simulink model "mainModelDoeJF"  (R2025a)
(part 2 of 3)

  heatGenModule16/1 -> SPC16/1
  heatGenModule17/1 -> SPC17/1
  heatGenModule18/1 -> SPC18/1
  heatGenModule19/1 -> SPC19/1
  heatGenModule20/1 -> SPC20/1
  heatGenModule21/1 -> SPC21/1
  heatGenModule22/1 -> SPC22/1
  heatGenModule23/1 -> SPC23/1
  heatGenModule24/1 -> SPC24/1
  heatGenModule25/1 -> SPC25/1
  heatGenModule26/1 -> SPC26/1
  heatGenModule27/1 -> SPC27/1
  heatGenModule28/1 -> SPC28/1
  heatGenModule29/1 -> SPC29/1
  heatGenModule30/1 -> SPC30/1
  heatGenModule31/1 -> SPC31/1
  heatGenModule32/1 -> SPC32/1
  TempProbeBlock1/1 -> thermalToElectricalConverter1/1  "T1"
  TempProbeBlock2/1 -> thermalToElectricalConverter2/1  "T2"
  TempProbeBlock3/1 -> thermalToElectricalConverter3/1  "T3"
  TempProbeBlock4/1 -> thermalToElectricalConverter4/1  "T4"
  TempProbeBlock5/1 -> thermalToElectricalConverter5/1  "T5"
  TempProbeBlock6/1 -> thermalToElectricalConverter6/1  "T6"
  TempProbeBlock7/1 -> thermalToElectricalConverter7/1  "T7"
  TempProbeBlock8/1 -> thermalToElectricalConverter8/1  "T8"
  TempProbeBlock9/1 -> thermalToElectricalConverter9/1  "T9"
  TempProbeBlock10/1 -> thermalToElectricalConverter10/1  "T10"
  TempProbeBlock11/1 -> thermalToElectricalConverter11/1  "T11"
  TempProbeBlock12/1 -> thermalToElectricalConverter12/1  "T12"
  TempProbeBlock13/1 -> thermalToElectricalConverter13/1  "T13"
  TempProbeBlock14/1 -> thermalToElectricalConverter14/1  "T14"
  TempProbeBlock15/1 -> thermalToElectricalConverter15/1  "T15"
  TempProbeBlock16/1 -> thermalToElectricalConverter16/1  "T16"
  TempProbeBlock17/1 -> thermalToElectricalConverter17/1  "T17"
  TempProbeBlock18/1 -> thermalToElectricalConverter18/1  "T18"
  TempProbeBlock19/1 -> thermalToElectricalConverter19/1  "T19"
  TempProbeBlock20/1 -> thermalToElectricalConverter20/1  "T20"
  TempProbeBlock21/1 -> thermalToElectricalConverter21/1  "T21"
  TempProbeBlock22/1 -> thermalToElectricalConverter22/1  "T22"
  TempProbeBlock23/1 -> thermalToElectricalConverter23/1  "T23"
  TempProbeBlock24/1 -> thermalToElectricalConverter24/1  "T24"
  TempProbeBlock25/1 -> thermalToElectricalConverter25/1  "T25"
  TempProbeBlock26/1 -> thermalToElectricalConverter26/1  "T26"
  TempProbeBlock27/1 -> thermalToElectricalConverter27/1  "T27"
  TempProbeBlock28/1 -> thermalToElectricalConverter28/1  "T28"
  TempProbeBlock29/1 -> thermalToElectricalConverter29/1  "T29"
  TempProbeBlock30/1 -> thermalToElectricalConverter30/1  "T30"
  TempProbeBlock31/1 -> thermalToElectricalConverter31/1  "T31"
  TempProbeBlock32/1 -> thermalToElectricalConverter32/1  "T32"
  connections:
  Module1/RConn1 -- Module2/LConn2
  Module2/RConn1 -- Module3/LConn2
  Module3/RConn1 -- Module4/LConn2
  Module4/RConn1 -- Module5/LConn2
  Module5/RConn1 -- Module6/LConn2
  Module6/RConn1 -- Module7/LConn2
  Module7/RConn1 -- Module8/LConn2
  Module8/RConn1 -- Module9/LConn2
  Module9/RConn1 -- Module10/LConn2
  Module10/RConn1 -- Module11/LConn2
  Module11/RConn1 -- Module12/LConn2
  Module12/RConn1 -- Module13/LConn2
  Module13/RConn1 -- Module14/LConn2
  Module14/RConn1 -- Module15/LConn2
  Module15/RConn1 -- Module16/LConn2
  Module16/RConn1 -- Module17/LConn2
  Module17/RConn1 -- Module18/LConn2
  Module18/RConn1 -- Module19/LConn2
  Module19/RConn1 -- Module20/LConn2
  Module20/RConn1 -- Module21/LConn2
  Module21/RConn1 -- Module22/LConn2
  Module22/RConn1 -- Module23/LConn2
  Module23/RConn1 -- Module24/LConn2
  Module24/RConn1 -- Module25/LConn2
  Module25/RConn1 -- Module26/LConn2
  Module26/RConn1 -- Module27/LConn2
  Module27/RConn1 -- Module28/LConn2
  Module28/RConn1 -- Module29/LConn2
  Module29/RConn1 -- Module30/LConn2
  Module30/RConn1 -- Module31/LConn2
  Module31/RConn1 -- Module32/LConn2
  Constant1/RConn1 -- Cycler/LConn3
  currentProfiletoSimscape/RConn1 -- Cycler/LConn1
  Cycler/RConn1 -- Module1/LConn2
  Cycler/RConn2 -- SolverConfig/RConn1 -- Module32/RConn1 -- ElectricalRef/LConn1
  coolantSwitchConverter/RConn1 -- coolantSwitchMultiplier/LConn2
  AdvectiveCoeff/RConn1 -- coolantSwitchMultiplier/LConn1
  CoolantCPCC1/LConn2 -- ThermalMassCPCC29/LConn1 -- TR_TMCPCC29/LConn1 -- CoolantBC1/LConn3
  CoolantCPCC1/LConn3 -- CoolantCPCC2/LConn2 -- ThermalMassCPCC30/LConn1 -- TR_TMCPCC30/LConn1
  CoolantCPCC1/LConn1 -- coolantSwitchMultiplier/RConn1 -- CoolantCPCC2/LConn1 -- CoolantCPCC3/LConn1 -- CoolantCPCC4/LConn1 -- CoolantCPCC5/LConn1 -- CoolantCPCC6/LConn1 -- CoolantCPCC7/LConn1 -- CoolantCPCC8/LConn1 -- CoolantCPCC9/LConn1 -- CoolantCPCC10/LConn1 -- CoolantCPCC11/LConn1 -- CoolantCPCC12/LConn1 -- CoolantCPCC13/LConn1 -- CoolantCPCC14/LConn1 -- CoolantCPCC15/LConn1 -- CoolantCPCC16/LConn1 -- CoolantCPCC17/LConn1 -- CoolantCPCC18/LConn1 -- CoolantCPCC19/LConn1 -- CoolantCPCC20/LConn1 -- CoolantCPCC21/LConn1 -- CoolantCPCC22/LConn1 -- CoolantCPCC23/LConn1 -- CoolantCPCC24/LConn1 -- CoolantCPCC25/LConn1 -- CoolantCPCC26/LConn1 -- CoolantCPCC27/LConn1 -- CoolantCPCC28/LConn1 -- CoolantCPCC29/LConn1 -- CoolantCPCC30/LConn1 -- CoolantCPCC31/LConn1 -- CoolantCPHC1/LConn1 -- CoolantCPHC2/LConn1 -- CoolantCPHC3/LConn1 -- CoolantCPHC4/LConn1 -- CoolantCPHC5/LConn1 -- CoolantCPHC6/LConn1 -- CoolantCPHC7/LConn1 -- CoolantCPHC8/LConn1 -- CoolantCPHC9/LConn1 -- CoolantCPHC10/LConn1 -- CoolantCPHC11/LConn1 -- CoolantCPHC12/LConn1 -- CoolantCPHC13/LConn1 -- CoolantCPHC14/LConn1 -- CoolantCPHC15/LConn1 -- CoolantCPHC16/LConn1 -- CoolantCPHC17/LConn1 -- CoolantCPHC18/LConn1 -- CoolantCPHC19/LConn1 -- CoolantCPHC20/LConn1 -- CoolantCPHC21/LConn1 -- CoolantCPHC22/LConn1 -- CoolantCPHC23/LConn1 -- CoolantCPHC24/LConn1 -- CoolantCPHC25/LConn1 -- CoolantCPHC26/LConn1 -- CoolantCPHC27/LConn1 -- CoolantCPHC28/LConn1 -- CoolantCPHC29/LConn1 -- CoolantCPHC30/LConn1 -- CoolantCPHC31/LConn1 -- CoolanthotCoolConnect63/LConn1 -- CoolantBC1/LConn1 -- CoolantBC2/LConn1
  CoolantCPCC2/LConn3 -- CoolantCPCC3/LConn2 -- ThermalMassCPCC31/LConn1 -- TR_TMCPCC31/LConn1
  CoolantCPCC3/LConn3 -- CoolantCPCC4/LConn2 -- ThermalMassCPCC32/LConn1 -- TR_TMCPCC32/LConn1
  CoolantCPCC4/LConn3 -- CoolantCPCC5/LConn2 -- ThermalMassCPCC4/LConn1 -- TR_TMCPCC4/LConn1
  CoolantCPCC5/LConn3 -- CoolantCPCC6/LConn2 -- ThermalMassCPCC3/LConn1 -- TR_TMCPCC3/LConn1
  CoolantCPCC6/LConn3 -- CoolantCPCC7/LConn2 -- ThermalMassCPCC2/LConn1 -- TR_TMCPCC2/LConn1
  CoolantCPCC7/LConn3 -- CoolantCPCC29/LConn2 -- ThermalMassCPCC1/LConn1 -- TR_TMCPCC1/LConn1
  CoolantCPCC8/LConn2 -- ThermalMassCPCC5/LConn1 -- CoolantCPCC29/LConn3 -- TR_TMCPCC5/LConn1
  CoolantCPCC8/LConn3 -- CoolantCPCC9/LConn2 -- ThermalMassCPCC6/LConn1 -- TR_TMCPCC6/LConn1
  CoolantCPCC9/LConn3 -- CoolantCPCC10/LConn2 -- ThermalMassCPCC7/LConn1 -- TR_TMCPCC7/LConn1
  CoolantCPCC10/LConn3 -- CoolantCPCC11/LConn2 -- ThermalMassCPCC8/LConn1 -- TR_TMCPCC8/LConn1
  CoolantCPCC11/LConn3 -- CoolantCPCC12/LConn2 -- ThermalMassCPCC28/LConn1 -- TR_TMCPCC28/LConn1
  CoolantCPCC12/LConn3 -- CoolantCPCC13/LConn2 -- ThermalMassCPCC27/LConn1 -- TR_TMCPCC27/LConn1
  CoolantCPCC13/LConn3 -- CoolantCPCC14/LConn2 -- ThermalMassCPCC26/LConn1 -- TR_TMCPCC26/LConn1
  CoolantCPCC14/LConn3 -- CoolantCPCC30/LConn2 -- ThermalMassCPCC25/LConn1 -- TR_TMCPCC25/LConn1
  CoolantCPCC15/LConn2 -- ThermalMassCPCC21/LConn1 -- CoolantCPCC30/LConn3 -- TR_TMCPCC21/LConn1
  CoolantCPCC15/LConn3 -- CoolantCPCC16/LConn2 -- ThermalMassCPCC22/LConn1 -- TR_TMCPCC22/LConn1
  CoolantCPCC16/LConn3 -- CoolantCPCC17/LConn2 -- ThermalMassCPCC23/LConn1 -- TR_TMCPCC23/LConn1
  CoolantCPCC17/LConn3 -- CoolantCPCC18/LConn2 -- ThermalMassCPCC24/LConn1 -- TR_TMCPCC24/LConn1
  CoolantCPCC18/LConn3 -- CoolantCPCC19/LConn2 -- ThermalMassCPCC12/LConn1 -- TR_TMCPCC12/LConn1
  CoolantCPCC19/LConn3 -- CoolantCPCC20/LConn2 -- ThermalMassCPCC11/LConn1 -- TR_TMCPCC11/LConn1
  CoolantCPCC20/LConn3 -- CoolantCPCC21/LConn2 -- ThermalMassCPCC10/LConn1 -- TR_TMCPCC10/LConn1
  CoolantCPCC21/LConn3 -- CoolantCPCC31/LConn2 -- ThermalMassCPCC9/LConn1 -- TR_TMCPCC9/LConn1
  CoolantCPCC22/LConn2 -- ThermalMassCPCC13/LConn1 -- CoolantCPCC31/LConn3 -- TR_TMCPCC13/LConn1
  CoolantCPCC22/LConn3 -- CoolantCPCC23/LConn2 -- ThermalMassCPCC14/LConn1 -- TR_TMCPCC14/LConn1
  CoolantCPCC23/LConn3 -- CoolantCPCC24/LConn2 -- ThermalMassCPCC15/LConn1 -- TR_TMCPCC15/LConn1
  CoolantCPCC24/LConn3 -- CoolantCPCC25/LConn2 -- ThermalMassCPCC16/LConn1 -- TR_TMCPCC16/LConn1
  CoolantCPCC25/LConn3 -- CoolantCPCC26/LConn2 -- ThermalMassCPCC20/LConn1 -- TR_TMCPCC20/LConn1
  CoolantCPCC26/LConn3 -- CoolantCPCC27/LConn2 -- ThermalMassCPCC19/LConn1 -- TR_TMCPCC19/LConn1
  CoolantCPCC27/LConn3 -- CoolantCPCC28/LConn2 -- ThermalMassCPCC18/LConn1 -- TR_TMCPCC18/LConn1
  CoolantCPCC28/LConn3 -- CoolanthotCoolConnect63/LConn2 -- ThermalMassCPCC17/LConn1 -- TR_TMCPCC17/LConn1
  CoolantCPHC1/LConn3 -- ThermalMassCPHC29/LConn1 -- TR_TMCPHC29/LConn1 -- CoolantBC2/LConn2
  CoolantCPHC1/LConn2 -- CoolantCPHC2/LConn3 -- ThermalMassCPHC30/LConn1 -- TR_TMCPHC30/LConn1
  CoolantCPHC2/LConn2 -- CoolantCPHC3/LConn3 -- ThermalMassCPHC31/LConn1 -- TR_TMCPHC31/LConn1
  CoolantCPHC3/LConn2 -- CoolantCPHC4/LConn3 -- ThermalMassCPHC32/LConn1 -- TR_TMCPHC32/LConn1
  CoolantCPHC4/LConn2 -- CoolantCPHC5/LConn3 -- ThermalMassCPHC4/LConn1 -- TR_TMCPHC4/LConn1
  CoolantCPHC5/LConn2 -- CoolantCPHC6/LConn3 -- ThermalMassCPHC3/LConn1 -- TR_TMCPHC3/LConn1
  CoolantCPHC6/LConn2 -- CoolantCPHC7/LConn3 -- ThermalMassCPHC2/LConn1 -- TR_TMCPHC2/LConn1
  CoolantCPHC7/LConn2 -- CoolantCPHC29/LConn3 -- ThermalMassCPHC1/LConn1 -- TR_TMCPHC1/LConn1
  CoolantCPHC8/LConn3 -- ThermalMassCPHC5/LConn1 -- CoolantCPHC29/LConn2 -- TR_TMCPHC5/LConn1
  CoolantCPHC8/LConn2 -- CoolantCPHC9/LConn3 -- ThermalMassCPHC6/LConn1 -- TR_TMCPHC6/LConn1
  CoolantCPHC9/LConn2 -- CoolantCPHC10/LConn3 -- ThermalMassCPHC7/LConn1 -- TR_TMCPHC7/LConn1
  CoolantCPHC10/LConn2 -- CoolantCPHC11/LConn3 -- ThermalMassCPHC8/LConn1 -- TR_TMCPHC8/LConn1
  CoolantCPHC11/LConn2 -- CoolantCPHC12/LConn3 -- ThermalMassCPHC28/LConn1 -- TR_TMCPHC28/LConn1
  CoolantCPHC12/LConn2 -- CoolantCPHC13/LConn3 -- ThermalMassCPHC27/LConn1 -- TR_TMCPHC27/LConn1
  CoolantCPHC13/LConn2 -- CoolantCPHC14/LConn3 -- ThermalMassCPHC26/LConn1 -- TR_TMCPHC26/LConn1
  CoolantCPHC14/LConn2 -- CoolantCPHC30/LConn3 -- ThermalMassCPHC25/LConn1 -- TR_TMCPHC25/LConn1
  CoolantCPHC15/LConn3 -- ThermalMassCPHC21/LConn1 -- CoolantCPHC30/LConn2 -- TR_TMCPHC21/LConn1
  CoolantCPHC15/LConn2 -- CoolantCPHC16/LConn3 -- ThermalMassCPHC22/LConn1 -- TR_TMCPHC22/LConn1
  CoolantCPHC16/LConn2 -- CoolantCPHC17/LConn3 -- ThermalMassCPHC23/LConn1 -- TR_TMCPHC23/LConn1
  CoolantCPHC17/LConn2 -- CoolantCPHC18/LConn3 -- ThermalMassCPHC24/LConn1 -- TR_TMCPHC24/LConn1
  CoolantCPHC18/LConn2 -- CoolantCPHC19/LConn3 -- ThermalMassCPHC12/LConn1 -- TR_TMCPHC12/LConn1
  CoolantCPHC19/LConn2 -- CoolantCPHC20/LConn3 -- ThermalMassCPHC11/LConn1 -- TR_TMCPHC11/LConn1
  CoolantCPHC20/LConn2 -- CoolantCPHC21/LConn3 -- ThermalMassCPHC10/LConn1 -- TR_TMCPHC10/LConn1
  CoolantCPHC21/LConn2 -- CoolantCPHC31/LConn3 -- ThermalMassCPHC9/LConn1 -- TR_TMCPHC9/LConn1
  CoolantCPHC22/LConn3 -- ThermalMassCPHC13/LConn1 -- CoolantCPHC31/LConn2 -- TR_TMCPHC13/LConn1
  CoolantCPHC22/LConn2 -- CoolantCPHC23/LConn3 -- ThermalMassCPHC14/LConn1 -- TR_TMCPHC14/LConn1
  CoolantCPHC23/LConn2 -- CoolantCPHC24/LConn3 -- ThermalMassCPHC15/LConn1 -- TR_TMCPHC15/LConn1
  CoolantCPHC24/LConn2 -- CoolantCPHC25/LConn3 -- ThermalMassCPHC16/LConn1 -- TR_TMCPHC16/LConn1
  CoolantCPHC25/LConn2 -- CoolantCPHC26/LConn3 -- ThermalMassCPHC20/LConn1 -- TR_TMCPHC20/LConn1
  CoolantCPHC26/LConn2 -- CoolantCPHC27/LConn3 -- ThermalMassCPHC19/LConn1 -- TR_TMCPHC19/LConn1
  CoolantCPHC27/LConn2 -- CoolantCPHC28/LConn3 -- ThermalMassCPHC18/LConn1 -- TR_TMCPHC18/LConn1
  CoolantCPHC28/LConn2 -- CoolanthotCoolConnect63/LConn3 -- ThermalMassCPHC17/LConn1 -- TR_TMCPHC17/LConn1
  TR_TMCPCC1/RConn1 -- TR_TMCPHC1/RConn1 -- TR_MA1/RConn1 -- ThermalMassBatteries1/LConn1 -- heat1/LConn1
  TR_TMCPCC2/RConn1 -- TR_TMCPHC2/RConn1 -- TR_MA2/RConn1 -- ThermalMassBatteries2/LConn1 -- heat2/LConn1
  TR_TMCPCC3/RConn1 -- TR_TMCPHC3/RConn1 -- TR_MA3/RConn1 -- ThermalMassBatteries3/LConn1 -- heat3/LConn1
  TR_TMCPCC4/RConn1 -- TR_TMCPHC4/RConn1 -- TR_MA4/RConn1 -- ThermalMassBatteries4/LConn1 -- heat4/LConn1
  TR_TMCPCC5/RConn1 -- TR_TMCPHC5/RConn1 -- TR_MA5/RConn1 -- ThermalMassBatteries5/LConn1 -- heat5/LConn1
  TR_TMCPCC6/RConn1 -- TR_TMCPHC6/RConn1 -- TR_MA6/RConn1 -- ThermalMassBatteries6/LConn1 -- heat6/LConn1
  TR_TMCPCC7/RConn1 -- TR_TMCPHC7/RConn1 -- TR_MA7/RConn1 -- ThermalMassBatteries7/LConn1 -- heat7/LConn1
  TR_TMCPCC8/RConn1 -- TR_TMCPHC8/RConn1 -- TR_MA8/RConn1 -- ThermalMassBatteries8/LConn1 -- heat8/LConn1
  TR_TMCPCC9/RConn1 -- TR_TMCPHC9/RConn1 -- TR_MA9/RConn1 -- ThermalMassBatteries9/LConn1 -- heat9/LConn1
  TR_TMCPCC10/RConn1 -- TR_TMCPHC10/RConn1 -- TR_MA10/RConn1 -- ThermalMassBatteries10/LConn1 -- heat10/LConn1
  TR_TMCPCC11/RConn1 -- TR_TMCPHC11/RConn1 -- TR_MA11/RConn1 -- ThermalMassBatteries11/LConn1 -- heat11/LConn1
  TR_TMCPCC12/RConn1 -- TR_TMCPHC12/RConn1 -- TR_MA12/RConn1 -- ThermalMassBatteries12/LConn1 -- heat12/LConn1
  TR_TMCPCC13/RConn1 -- TR_TMCPHC13/RConn1 -- TR_MA13/RConn1 -- ThermalMassBatteries13/LConn1 -- heat13/LConn1
  TR_TMCPCC14/RConn1 -- TR_TMCPHC14/RConn1 -- TR_MA14/RConn1 -- ThermalMassBatteries14/LConn1 -- heat14/LConn1
  TR_TMCPCC15/RConn1 -- TR_TMCPHC15/RConn1 -- TR_MA15/RConn1 -- ThermalMassBatteries15/LConn1 -- heat15/LConn1
  TR_TMCPCC16/RConn1 -- TR_TMCPHC16/RConn1 -- TR_MA16/RConn1 -- ThermalMassBatteries16/LConn1 -- heat16/LConn1
  TR_TMCPCC17/RConn1 -- TR_TMCPHC17/RConn1 -- TR_MA17/RConn1 -- ThermalMassBatteries17/LConn1 -- heat17/LConn1
  TR_TMCPCC18/RConn1 -- TR_TMCPHC18/RConn1 -- TR_MA18/RConn1 -- ThermalMassBatteries18/LConn1 -- heat18/LConn1
  TR_TMCPCC19/RConn1 -- TR_TMCPHC19/RConn1 -- TR_MA19/RConn1 -- ThermalMassBatteries19/LConn1 -- heat19/LConn1
  TR_TMCPCC20/RConn1 -- TR_TMCPHC20/RConn1 -- TR_MA20/RConn1 -- ThermalMassBatteries20/LConn1 -- heat20/LConn1
  TR_TMCPCC21/RConn1 -- TR_TMCPHC21/RConn1 -- TR_MA21/RConn1 -- ThermalMassBatteries21/LConn1 -- heat21/LConn1
  TR_TMCPCC22/RConn1 -- TR_TMCPHC22/RConn1 -- TR_MA22/RConn1 -- ThermalMassBatteries22/LConn1 -- heat22/LConn1
  TR_TMCPCC23/RConn1 -- TR_TMCPHC23/RConn1 -- TR_MA23/RConn1 -- ThermalMassBatteries23/LConn1 -- heat23/LConn1
  TR_TMCPCC24/RConn1 -- TR_TMCPHC24/RConn1 -- TR_MA24/RConn1 -- ThermalMassBatteries24/LConn1 -- heat24/LConn1
  TR_TMCPCC25/RConn1 -- TR_TMCPHC25/RConn1 -- TR_MA25/RConn1 -- ThermalMassBatteries25/LConn1 -- heat25/LConn1
  TR_TMCPCC26/RConn1 -- TR_TMCPHC26/RConn1 -- TR_MA26/RConn1 -- ThermalMassBatteries26/LConn1 -- heat26/LConn1
  TR_TMCPCC27/RConn1 -- TR_TMCPHC27/RConn1 -- TR_MA27/RConn1 -- ThermalMassBatteries27/LConn1 -- heat27/LConn1
  TR_TMCPCC28/RConn1 -- TR_TMCPHC28/RConn1 -- TR_MA28/RConn1 -- ThermalMassBatteries28/LConn1 -- heat28/LConn1
  TR_TMCPCC29/RConn1 -- TR_TMCPHC29/RConn1 -- TR_MA29/RConn1 -- ThermalMassBatteries29/LConn1 -- heat29/LConn1
  TR_TMCPCC30/RConn1 -- TR_TMCPHC30/RConn1 -- TR_MA30/RConn1 -- ThermalMassBatteries30/LConn1 -- heat30/LConn1
  TR_TMCPCC31/RConn1 -- TR_TMCPHC31/RConn1 -- TR_MA31/RConn1 -- ThermalMassBatteries31/LConn1 -- heat31/LConn1
  TR_TMCPCC32/RConn1 -- TR_TMCPHC32/RConn1 -- TR_MA32/RConn1 -- ThermalMassBatteries32/LConn1 -- heat32/LConn1
  TempSource/RConn2 -- ThermalReference/LConn1 -- heat1/RConn2 -- heat2/RConn2 -- heat3/RConn2 -- heat4/RConn2 -- heat5/RConn2 -- heat6/RConn2 -- heat7/RConn2 -- heat8/RConn2 -- heat9/RConn2 -- heat10/RConn2 -- heat11/RConn2 -- heat12/RConn2 -- heat13/RConn2 -- heat14/RConn2 -- heat15/RConn2 -- heat16/RConn2 -- heat17/RConn2 -- heat18/RConn2 -- heat19/RConn2 -- heat20/RConn2 -- heat21/RConn2 -- heat22/RConn2 -- heat23/RConn2 -- heat24/RConn2 -- heat25/RConn2 -- heat26/RConn2 -- heat27/RConn2 -- heat28/RConn2 -- heat29/RConn2 -- heat30/RConn2 -- heat31/RConn2 -- heat32/RConn2 -- ThermalSolverConfig/RConn1
  ConstantTemp/RConn1 -- TempSource/RConn1
  TR_MA1/LConn1 -- TempSource/LConn1 -- TR_MA2/LConn1 -- TR_MA3/LConn1 -- TR_MA4/LConn1 -- TR_MA5/LConn1 -- TR_MA6/LConn1 -- TR_MA7/LConn1 -- TR_MA8/LConn1 -- TR_MA9/LConn1 -- TR_MA10/LConn1 -- TR_MA11/LConn1 -- TR_MA12/LConn1 -- TR_MA13/LConn1 -- TR_MA14/LConn1 -- TR_MA15/LConn1 -- TR_MA16/LConn1 -- TR_MA17/LConn1 -- TR_MA18/LConn1 -- TR_MA19/LConn1 -- TR_MA20/LConn1 -- TR_MA21/LConn1 -- TR_MA22/LConn1 -- TR_MA23/LConn1 -- TR_MA24/LConn1 -- TR_MA25/LConn1 -- TR_MA26/LConn1 -- TR_MA27/LConn1 -- TR_MA28/LConn1 -- TR_MA29/LConn1 -- TR_MA30/LConn1 -- TR_MA31/LConn1 -- TR_MA32/LConn1
  CoolantTempSource/LConn1 -- CoolantBC1/LConn2 -- CoolantBC2/LConn3
  SPC1/RConn1 -- heat1/RConn1
  SPC2/RConn1 -- heat2/RConn1
  SPC3/RConn1 -- heat3/RConn1
  SPC4/RConn1 -- heat4/RConn1
  SPC5/RConn1 -- heat5/RConn1
  SPC6/RConn1 -- heat6/RConn1
  SPC7/RConn1 -- heat7/RConn1
  SPC8/RConn1 -- heat8/RConn1
  SPC9/RConn1 -- heat9/RConn1
  SPC10/RConn1 -- heat10/RConn1
  SPC11/RConn1 -- heat11/RConn1
  SPC12/RConn1 -- heat12/RConn1
  SPC13/RConn1 -- heat13/RConn1
  SPC14/RConn1 -- heat14/RConn1
  SPC15/RConn1 -- heat15/RConn1
  SPC16/RConn1 -- heat16/RConn1
  SPC17/RConn1 -- heat17/RConn1
  SPC18/RConn1 -- heat18/RConn1
  SPC19/RConn1 -- heat19/RConn1
  SPC20/RConn1 -- heat20/RConn1
  SPC21/RConn1 -- heat21/RConn1
  SPC22/RConn1 -- heat22/RConn1
  SPC23/RConn1 -- heat23/RConn1
  SPC24/RConn1 -- heat24/RConn1
  SPC25/RConn1 -- heat25/RConn1
  SPC26/RConn1 -- heat26/RConn1
  SPC27/RConn1 -- heat27/RConn1
  SPC28/RConn1 -- heat28/RConn1
  SPC29/RConn1 -- heat29/RConn1
  SPC30/RConn1 -- heat30/RConn1
  SPC31/RConn1 -- heat31/RConn1
  SPC32/RConn1 -- heat32/RConn1
  tempSource1/RConn2 -- ThermalReferenceInElectricalModel/LConn1 -- tempSource2/RConn2 -- tempSource3/RConn2 -- tempSource4/RConn2 -- tempSource5/RConn2 -- tempSource6/RConn2 -- tempSource7/RConn2 -- tempSource8/RConn2 -- tempSource9/RConn2 -- tempSource10/RConn2 -- tempSource11/RConn2 -- tempSource12/RConn2 -- tempSource13/RConn2 -- tempSource14/RConn2 -- tempSource15/RConn2 -- tempSource16/RConn2 -- tempSource17/RConn2 -- tempSource18/RConn2 -- tempSource19/RConn2 -- tempSource20/RConn2 -- tempSource21/RConn2 -- tempSource22/RConn2 -- tempSource23/RConn2 -- tempSource24/RConn2 -- tempSource25/RConn2 -- tempSource26/RConn2 -- tempSource27/RConn2 -- tempSource28/RConn2 -- tempSource29/RConn2 -- tempSource30/RConn2 -- tempSource31/RConn2 -- tempSource32/RConn2
  tempSource1/LConn1 -- Module1/LConn1
  thermalToElectricalConverter1/RConn1 -- tempSource1/RConn1
  tempSource2/LConn1 -- Module2/LConn1
  thermalToElectricalConverter2/RConn1 -- tempSource2/RConn1
  tempSource3/LConn1 -- Module3/LConn1
  thermalToElectricalConverter3/RConn1 -- tempSource3/RConn1
  tempSource4/LConn1 -- Module4/LConn1
  thermalToElectricalConverter4/RConn1 -- tempSource4/RConn1
  tempSource5/LConn1 -- Module5/LConn1
  thermalToElectricalConverter5/RConn1 -- tempSource5/RConn1
  tempSource6/LConn1 -- Module6/LConn1
  thermalToElectricalConverter6/RConn1 -- tempSource6/RConn1
  tempSource7/LConn1 -- Module7/LConn1
  thermalToElectricalConverter7/RConn1 -- tempSource7/RConn1
  tempSource8/LConn1 -- Module8/LConn1
  thermalToElectricalConverter8/RConn1 -- tempSource8/RConn1
  tempSource9/LConn1 -- Module9/LConn1
  thermalToElectricalConverter9/RConn1 -- tempSource9/RConn1
  tempSource10/LConn1 -- Module10/LConn1
  thermalToElectricalConverter10/RConn1 -- tempSource10/RConn1
  tempSource11/LConn1 -- Module11/LConn1
  thermalToElectricalConverter11/RConn1 -- tempSource11/RConn1
  tempSource12/LConn1 -- Module12/LConn1
  thermalToElectricalConverter12/RConn1 -- tempSource12/RConn1
  tempSource13/LConn1 -- Module13/LConn1
  thermalToElectricalConverter13/RConn1 -- tempSource13/RConn1
  tempSource14/LConn1 -- Module14/LConn1
  thermalToElectricalConverter14/RConn1 -- tempSource14/RConn1
  tempSource15/LConn1 -- Module15/LConn1
  thermalToElectricalConverter15/RConn1 -- tempSource15/RConn1
  tempSource16/LConn1 -- Module16/LConn1
  thermalToElectricalConverter16/RConn1 -- tempSource16/RConn1
  tempSource17/LConn1 -- Module17/LConn1
  thermalToElectricalConverter17/RConn1 -- tempSource17/RConn1
  tempSource18/LConn1 -- Module18/LConn1
  thermalToElectricalConverter18/RConn1 -- tempSource18/RConn1
  tempSource19/LConn1 -- Module19/LConn1
  thermalToElectricalConverter19/RConn1 -- tempSource19/RConn1
  tempSource20/LConn1 -- Module20/LConn1
  thermalToElectricalConverter20/RConn1 -- tempSource20/RConn1
  tempSource21/LConn1 -- Module21/LConn1
  thermalToElectricalConverter21/RConn1 -- tempSource21/RConn1
  tempSource22/LConn1 -- Module22/LConn1
  thermalToElectricalConverter22/RConn1 -- tempSource22/RConn1
  tempSource23/LConn1 -- Module23/LConn1
  thermalToElectricalConverter23/RConn1 -- tempSource23/RConn1
  tempSource24/LConn1 -- Module24/LConn1
  thermalToElectricalConverter24/RConn1 -- tempSource24/RConn1
  tempSource25/LConn1 -- Module25/LConn1
  thermalToElectricalConverter25/RConn1 -- tempSource25/RConn1
  tempSource26/LConn1 -- Module26/LConn1
  thermalToElectricalConverter26/RConn1 -- tempSource26/RConn1
  tempSource27/LConn1 -- Module27/LConn1
  thermalToElectricalConverter27/RConn1 -- tempSource27/RConn1
  tempSource28/LConn1 -- Module28/LConn1
  thermalToElectricalConverter28/RConn1 -- tempSource28/RConn1
  tempSource29/LConn1 -- Module29/LConn1
  thermalToElectricalConverter29/RConn1 -- tempSource29/RConn1
  tempSource30/LConn1 -- Module30/LConn1
  thermalToElectricalConverter30/RConn1 -- tempSource30/RConn1
  tempSource31/LConn1 -- Module31/LConn1
  thermalToElectricalConverter31/RConn1 -- tempSource31/RConn1
  tempSource32/LConn1 -- Module32/LConn1
  thermalToElectricalConverter32/RConn1 -- tempSource32/RConn1
